simulink model "robotarm_generalization_error"  (R2018b)
settings: Solver=FixedStepAuto  StartTime=0.0  StopTime=10  FixedStep=options.dt  RelTol=1e-3  AbsTol=1e-6
PreLoadFcn:
  | const_ref=-0.1;
  | options.dt=0.02;
libraries: neural x528, simulink x1
(part 20 of 20)

== system robotarm_generalization_error/pre_0.01/Layer 3/Delays 1 ==
  "p{3}" : Inport  PortDimensions=30
      mask Display: e = 0.06;c1 = [120 230 180]/255;c2 = ([120 230 180]+0)/(256+128);c3 = ([120 230 180]+128)/(256+128);patch([0 1 1 0],[0 0 1 1],c1);patch([0 1 1 1-e 1-e 0+e],[0 0 1 1-e 0+e 0+e],c2);patch([0 0 1 1-e 0+e 0+e],[0 1 1 1-e 1-e 0+e],c3);plot([0 1 1 0 0],[0 0 1 1 0]);
  mux : Mux  Inputs=1
      mask Display: e = 0.06;c1 = [120 150 230]/255;c2 = ([120 150 230]+0)/383;c3 = ([120 150 230]+128)/383;patch([0 1 1 0],[0 0 1 1],c1);patch([0 1 1 1-e 1-e 0+e],[0 0 1 1-e 0+e 0+e],c2);patch([0 0 1 1-e 0+e 0+e],[0 1 1 1-e 1-e 0+e],c3);plot([0 1 1 0 0],[0 0 1 1 0]);disp('Mux')
  "pd{3,2}" : Outport
      mask Display: e = 0.06;c1 = [120 230 180]/255;c2 = ([120 230 180]+0)/(256+128);c3 = ([120 230 180]+128)/(256+128);patch([0 1 1 0],[0 0 1 1],c1);patch([0 1 1 1-e 1-e 0+e],[0 0 1 1-e 0+e 0+e],c2);patch([0 0 1 1-e 0+e 0+e],[0 1 1 1-e 1-e 0+e],c3);plot([0 1 1 0 0],[0 0 1 1 0]);
  wires:
  "p{3}"/1 -> mux/1
  mux/1 -> "pd{3,2}"/1

== system robotarm_generalization_error/pre_0.01/Layer 3/LW{3,2} ==
  "ad{3,2}" : Inport  PortDimensions=30
      mask Display: e = 0.06;c1 = [120 230 180]/255;c2 = ([120 230 180]+0)/(256+128);c3 = ([120 230 180]+128)/(256+128);patch([0 1 1 0],[0 0 1 1],c1);patch([0 1 1 1-e 1-e 0+e],[0 0 1 1-e 0+e 0+e],c2);patch([0 0 1 1-e 0+e 0+e],[0 1 1 1-e 1-e 0+e],c3);plot([0 1 1 0 0],[0 0 1 1 0]);
  "IW{3,2}(1,:)'" : Constant  Value=[-0.0729389813017181920518083870774717070162296295166015625;-0.002015841098917082845065618101898508029989898204803466796875;0.068032878692783460561344099915004335343837738037109375;-0.039155678019892968533266497388467541895806789398193359375;-0.0210182537300655537804150441161255002953112125396728515625;-0.0989324868727098627463334423737251199781894683837890625;0.042928551049714970544446401845561922527849674224853515625;0.0082298165636691920921119702825308195315301418304443359375;0.007028176883428623351879327429969634977169334888458251953125;-0.035382315048845210114780712729043443687260150909423828125;-0.08894534648935605025688033720143721438944339752197265625;0.017505008899830955260146225782591500319540500640869140625;0.04004596619473192731231137031500111334025859832763671875;-0.04855976328719645296327911410116939805448055267333984375;-0.01599486508337945311897243527710088528692722320556640625;-0.033110409861825777777522006317667546682059764862060546875;0.01992223693813761908888437801579129882156848907470703125;0.00767285991208370606042610262420566868968307971954345703125;-0.0155743215435539157642796936897866544313728809356689453125;-0.046790695776373243675028135157845099456608295440673828125;-0.02122592592859968985141705388741684146225452423095703125;0.017191426900235208530265396120739751495420932769775390625;0.052081926000509627672219181704349466599524021148681640625;-0.005394369041407645094798883889097851351834833621978759765625;-0.002320895426048841074517792293363527278415858745574951171875;-0.032398862638842097771973982389681623317301273345947265625;-0.02497692721570081431092802404236863367259502410888671875;-0.033123993786144188822273548566954559646546840667724609375;-0.038305265753547701468306740935076959431171417236328125;-0.04083860284675623619765616467702784575521945953369140625]
      mask Display: e = 0.06;c1 = [120 150 230]/255;c2 = ([120 150 230]+0)/383;c3 = ([120 150 230]+128)/383;patch([0 1 1 0],[0 0 1 1],c1);patch([0 1 1 1-e 1-e 0+e],[0 0 1 1-e 0+e 0+e],c2);patch([0 0 1 1-e 0+e 0+e],[0 1 1 1-e 1-e 0+e],c3);plot([0 1 1 0 0],[0 0 1 1 0]);disp('weights');
  Mux : Mux  Inputs=1
      mask Display: e = 0.06;c1 = [120 150 230]/255;c2 = ([120 150 230]+0)/383;c3 = ([120 150 230]+128)/383;patch([0 1 1 0],[0 0 1 1],c1);patch([0 1 1 1-e 1-e 0+e],[0 0 1 1-e 0+e 0+e],c2);patch([0 0 1 1-e 0+e 0+e],[0 1 1 1-e 1-e 0+e],c3);plot([0 1 1 0 0],[0 0 1 1 0]);disp('Mux');
  dotprod1 : neural/Weight Functions/dotprod
  "lz{3,2}" : Outport
      mask Display: e = 0.06;c1 = [120 230 180]/255;c2 = ([120 230 180]+0)/(256+128);c3 = ([120 230 180]+128)/(256+128);patch([0 1 1 0],[0 0 1 1],c1);patch([0 1 1 1-e 1-e 0+e],[0 0 1 1-e 0+e 0+e],c2);patch([0 0 1 1-e 0+e 0+e],[0 1 1 1-e 1-e 0+e],c3);plot([0 1 1 0 0],[0 0 1 1 0]);
  wires:
  "IW{3,2}(1,:)'"/1 -> dotprod1/1
  "ad{3,2}"/1 -> dotprod1/2
  dotprod1/1 -> Mux/1
  Mux/1 -> "lz{3,2}"/1
